simulink model "Experiment_AERO_pitch_channel_identification"  (Simulink 9.1)
settings: Solver=ode4  StartTime=0.0  StopTime=30  FixedStep=0.001  RelTol=1e-3  EnableMultiTasking=on
InitFcn:
  | Parameters_and_initial_conditions
values from neighbouring files (symbols this model uses):
  Dp = 0.0056    [Parameters_and_initial_conditions.m]    (also in quanser_aero_parameters.m = 0.0071116)
  Dy = 0.0220    (= 0.022)    [Parameters_and_initial_conditions.m]    (also in quanser_aero_parameters.m)
  Jp = J_body + 2*J_prop    (= 0.0218868648283)    [Parameters_and_initial_conditions.m]    (also in quanser_aero_parameters.m)
  Jy = J_body + 2*J_prop + J_yoke    (= 0.0219920648283)    [Parameters_and_initial_conditions.m]    (also in quanser_aero_parameters.m)
  Kpp = 10.9e-04    (= 0.00109)    [Parameters_and_initial_conditions.m]    (also in quanser_aero_parameters.m = 0.0011)
  Kpy = 0.0021    [Parameters_and_initial_conditions.m]    (also in quanser_aero_parameters.m)
  Ksp = 0.09    [Parameters_and_initial_conditions.m]    (also in quanser_aero_parameters.m = 0.037463)
  Kyp = -0.0027    [Parameters_and_initial_conditions.m]    (also in quanser_aero_parameters.m)
  Kyy = 0.0022    [Parameters_and_initial_conditions.m]    (also in quanser_aero_parameters.m)
  PitchAxisEnable = 1    [Parameters_and_initial_conditions.m]
  PitchMotorEnable = 1    [Parameters_and_initial_conditions.m]
  psi_dot_initial = 0.0    (= 0)    [Parameters_and_initial_conditions.m]
  psi_initial = 0.0    (= 0)    [Parameters_and_initial_conditions.m]
  theta_dot_initial = 0.0    (= 0)    [Parameters_and_initial_conditions.m]
  theta_initial = 0.0    (= 0)    [Parameters_and_initial_conditions.m]
  YawAxisEnable = 0    [Parameters_and_initial_conditions.m]
  YawMotorEnable = 0    [Parameters_and_initial_conditions.m]
libraries: quarc_library x7, simulink_extras x5, quanser_aero x1
settings Model: Creator=MLevis  LastModifiedBy=DELL  SimulationMode=external  ExtModeTrigDuration=5000
settings SolverCC: PositivePriorityOrder=on
settings DataIOCC: LimitDataPoints=on
settings DebuggingCC: UnderspecifiedInitializationDetection=Simplified  MergeDetectMultiDrivingBlocksExec=error  SolverPrmCheckMsg=warning
settings RTWCC: SystemTargetFile=quarc_win64.tlc  TemplateMakefile=quarc_default_tmf  Description=QUARC Win64 Target
settings STFCustomTargetCC: TargetPreCompLibLocation=C:\PROGRA~3\QUARC\lib\2018a\win64\release  ConcurrentExecutionCompliant=on  GeneratePreprocessorConditionals=Disable all  SystemTargetFile=quarc_win64.tlc
settings GRTTargetCC: TargetPreCompLibLocation=C:\PROGRA~3\QUARC\lib\2018a\win64\release  ParMdlRefBuildCompliant=off  CompOptLevelCompliant=off  GeneratePreprocessorConditionals=Disable all  MatFileLogging=off  CPPClassGenCompliant=off  UseToolchainInfoCompliant=off  ExtMode=on  ExtModeMexFile=quarc_comm
settings ConfigComp: CovSFcnEnable=off

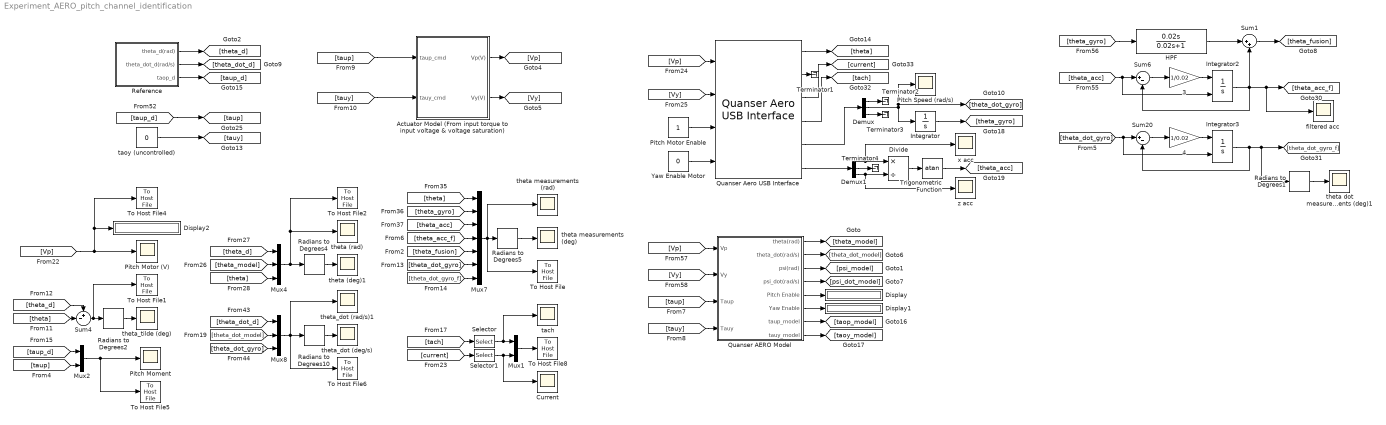
== system Experiment_AERO_pitch_channel_identification ==
  " 3" : Gain  Gain=1/0.02
  " 4" : Gain  Gain=1/0.02
  Actuator Model (From input torque to input voltage & voltage saturation) : Subsystem
  Current : Scope
  Demux : Demux  Outputs=3
  Demux1 : Demux  Outputs=3
  Display : Display
  Display1 : Display
  Display2 : Display
  Divide : Product  Inputs=*/
  HPF : TransferFcn  Numerator=[0.02 0]  Denominator=[0.02 1]
  Integrator : Integrator
  Integrator2 : Integrator  InitialConditionSource=external
  Integrator3 : Integrator  InitialConditionSource=external
  Mux1 : Mux  Inputs=2
  Mux2 : Mux  Inputs=2
  Mux4 : Mux  Inputs=3
  Mux7 : Mux  Inputs=7
  Mux8 : Mux  Inputs=3
  Pitch Moment : Scope
  Pitch Motor (V) : Scope
  Pitch Motor Enable : Constant
  Pitch Speed (rad/s) : Scope
  Quanser AERO Model : Subsystem
  Quanser Aero USB Interface : quanser_aero/Quanser Aero USB Interface
  Radians to Degrees{1..2,4..5,10} (5 alike) : simulink_extras/Transformations/Radians to Degrees
  Reference : Subsystem
  Selector : Selector  InputPortWidth=2  IndexOptions=Index vector (dialog)  Indices=[1]  OutputSizes=1
  Selector1 : Selector  InputPortWidth=2  IndexOptions=Index vector (dialog)  Indices=[1]  OutputSizes=1
  Sum1 : Sum  Inputs=|++
  Sum20 : Sum  Inputs=|+-
  Sum4 : Sum  Inputs=+-|
  Sum6 : Sum  Inputs=|+-
  Terminator{1..4} (4 alike) : Terminator
  To Host File : quarc_library/Sinks/To Host/To Host File  file_name=Log_Sensor_Measurements.mat  variable_name=Log_Sensor_Measurements  decimation=1  sample_time=-1  file_format=MAT-file v.5  options=No header or footer  append=off  final_file_name=Log_Sensor_Measurements.mat  bitrate=2000000
  To Host File1 : quarc_library/Sinks/To Host/To Host File  file_name=Log_Tracking_Err.mat  variable_name=Log_Tracking_Err  decimation=1  sample_time=-1  file_format=MAT-file v.5  options=No header or footer  append=off  final_file_name=Log_Tracking_Err.mat  bitrate=2000000
  To Host File2 : quarc_library/Sinks/To Host/To Host File  file_name=Log_Theta_Response.mat  variable_name=Log_Theta_Response  decimation=1  sample_time=-1  file_format=MAT-file v.5  options=No header or footer  append=off  final_file_name=Log_Theta_Response.mat  bitrate=2000000
  To Host File4 : quarc_library/Sinks/To Host/To Host File  file_name=Log_Input_Voltage.mat  variable_name=Log_Input_Voltage  decimation=1  sample_time=-1  file_format=MAT-file v.5  options=No header or footer  append=off  final_file_name=Log_Input_Voltage.mat  bitrate=2000000
  To Host File5 : quarc_library/Sinks/To Host/To Host File  file_name=Log_Input_Torque.mat  variable_name=Log_Input_Torque  decimation=1  sample_time=-1  file_format=MAT-file v.5  options=No header or footer  append=off  final_file_name=Log_Input_Torque.mat  bitrate=2000000
  To Host File6 : quarc_library/Sinks/To Host/To Host File  file_name=Log_Theta_dot_Response.mat  variable_name=Log_Theta_dot_Response  decimation=1  sample_time=-1  file_format=MAT-file v.5  options=No header or footer  append=off  final_file_name=Log_Theta_dot_Response.mat  bitrate=2000000
  To Host File8 : quarc_library/Sinks/To Host/To Host File  file_name=Log_Tach_Current.mat  variable_name=Log_Tach_Current  decimation=1  sample_time=-1  file_format=MAT-file v.5  options=No header or footer  append=off  final_file_name=Log_Tach_Current.mat  bitrate=2000000
  Trigonometric Function : Trigonometry  Operator=atan
  Yaw Enable Motor : Constant  Value=0
  filtered acc : Scope
  tach : Scope
  taoy (uncontrolled) : Constant  Value=0
  theta (deg)1 : Scope
  theta (rad) : Scope
  theta dot measurements (deg)1 : Scope
  theta measurements (deg) : Scope
  theta measurements (rad) : Scope
  theta_dot (deg/s) : Scope
  theta_dot (rad/s)1 : Scope
  theta_tilde (deg) : Scope
  x acc : Scope
  z acc : Scope
  wires:
  Quanser AERO Model/3(psi(rad)) -> [psi_model]
  Quanser AERO Model/1(theta(rad)) -> [theta_model]
  Reference/1(theta_d(rad)) -> [theta_d]
  Quanser AERO Model/2(theta_dot(rad/s)) -> [theta_dot_model]
  Quanser AERO Model/4(psi_dot(rad/s)) -> [psi_dot_model]
  Quanser AERO Model/5(Pitch Enable) -> Display/1
  Quanser AERO Model/6(Yaw Enable) -> Display1/1
  Actuator Model (From input torque to input voltage & voltage saturation)/1(Vp(V)) -> [Vp]
  Actuator Model (From input torque to input voltage & voltage saturation)/2(Vy(V)) -> [Vy]
  [tauy] -> Actuator Model (From input torque to input voltage & voltage saturation)/2(tauy_cmd)
  [taup] -> Actuator Model (From input torque to input voltage & voltage saturation)/1(taup_cmd)
  [theta_d] -> Sum4/1
  [theta] -> Sum4/2
  Sum4/1 -> To Host File1/1, Radians to Degrees2/1
  Radians to Degrees2/1 -> theta_tilde (deg)/1
  Reference/2(theta_dot_d(rad/s)) -> [theta_dot_d]
  Reference/3(taop_d) -> [taup_d]
  [taup] -> Mux2/2
  [taup_d] -> Mux2/1
  taoy (uncontrolled)/1 -> [tauy]
  [Vp] -> To Host File4/1, Display2/1, Pitch Motor (V)/1
  Quanser Aero USB Interface/5 -> Demux/1
  Yaw Enable Motor/1 -> Quanser Aero USB Interface/4
  Quanser Aero USB Interface/4 -> [tach]
  Quanser Aero USB Interface/1 -> [theta]
  Demux/3 -> Terminator3/1
  Pitch Motor Enable/1 -> Quanser Aero USB Interface/3
  Quanser Aero USB Interface/3 -> [current]
  [Vy] -> Quanser Aero USB Interface/2
  Demux/1 -> Terminator2/1
  Demux/2 -> Pitch Speed (rad/s)/1, [theta_dot_gyro], Integrator/1
  Quanser Aero USB Interface/2 -> Terminator1/1
  Quanser Aero USB Interface/6 -> Demux1/1
  [Vp] -> Quanser Aero USB Interface/1
  Radians to Degrees4/1 -> theta (deg)1/1
  [theta_model] -> Mux4/2
  [theta_d] -> Mux4/1
  [theta] -> Mux4/3
  Quanser AERO Model/7(taup_model) -> [taop_model]
  Mux2/1 -> To Host File5/1, Pitch Moment/1
  Quanser AERO Model/8(tauy_model) -> [taoy_model]
  Integrator/1 -> [theta_gyro]
  [theta] -> Mux7/1
  Demux1/1 -> Divide/1, x acc/1
  Demux1/2 -> Terminator4/1
  Demux1/3 -> Divide/2, z acc/1
  Divide/1 -> Trigonometric Function/1
  Trigonometric Function/1 -> [theta_acc]
  [theta_gyro] -> Mux7/2
  [theta_acc] -> Mux7/3
  Radians to Degrees5/1 -> theta measurements (deg)/1
  Radians to Degrees10/1 -> theta_dot (deg/s)/1
  [theta_dot_model] -> Mux8/2
  Mux8/1 -> theta_dot (rad/s)1/1, To Host File6/1, Radians to Degrees10/1
  [theta_dot_gyro] -> Mux8/3
  [theta_dot_d] -> Mux8/1
  [theta_gyro] -> HPF/1
  HPF/1 -> Sum1/1
  Sum1/1 -> [theta_fusion]
  [theta_acc_f] -> Mux7/4
  Mux7/1 -> theta measurements (rad)/1, To Host File/1, Radians to Degrees5/1
  [taup] -> Quanser AERO Model/3(Taup)
  [tauy] -> Quanser AERO Model/4(Tauy)
  [Vp] -> Quanser AERO Model/1(Vp)
  [Vy] -> Quanser AERO Model/2(Vy)
  [taup_d] -> [taup]
  Mux4/1 -> Radians to Degrees4/1, To Host File2/1, theta (rad)/1
  Integrator2/1 -> Sum1/2, Sum6/2, filtered acc/1, [theta_acc_f]
  " 3"/1 -> Integrator2/1
  Sum6/1 -> " 3"/1
  [theta_acc] -> Integrator2/2, Sum6/1
  [theta_fusion] -> Mux7/5
  [theta_dot_gyro] -> Integrator3/2, Sum20/1
  Sum20/1 -> " 4"/1
  " 4"/1 -> Integrator3/1
  Integrator3/1 -> Radians to Degrees1/1, [theta_dot_gyro_f], Sum20/2
  Radians to Degrees1/1 -> theta dot measurements (deg)1/1
  [theta_dot_gyro] -> Mux7/6
  [theta_dot_gyro_f] -> Mux7/7
  [tach] -> Selector/1
  Mux1/1 -> To Host File8/1
  [current] -> Selector1/1
  Selector/1 -> tach/1, Mux1/1
  Selector1/1 -> Current/1, Mux1/2

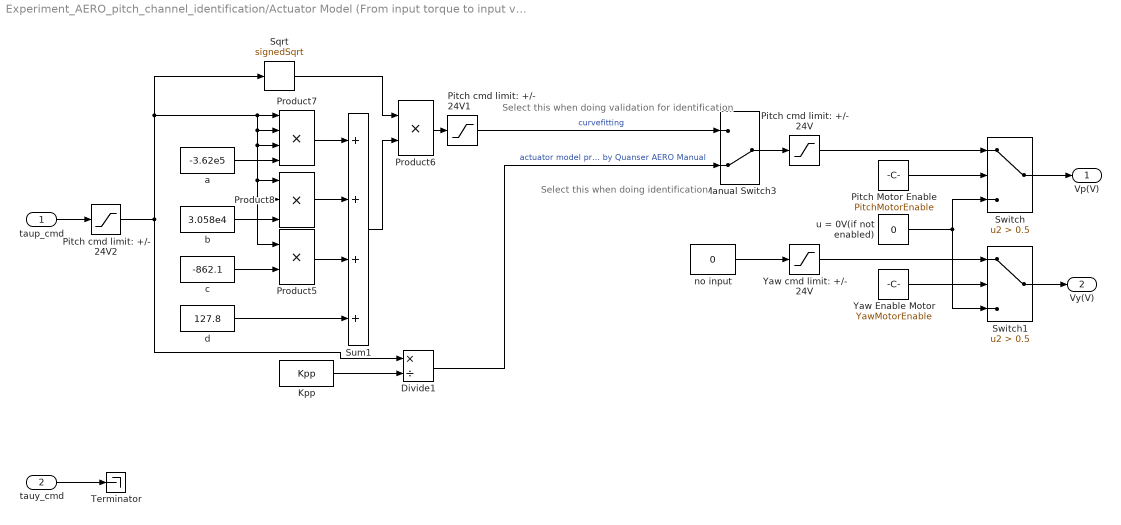
== system Experiment_AERO_pitch_channel_identification/Actuator Model (From input torque to input voltage & voltage saturation) ==
  note: Select this when doing identification
  note: Select this when doing validation for identification
  taup_cmd : Inport
  tauy_cmd : Inport  Port=2
  Divide1 : Product  Inputs=*/
  Kpp : Constant  Value=Kpp
  Manual Switch3 : ManualSwitch  CurrentSetting=0
  Pitch Motor Enable : Constant  Value=PitchMotorEnable
  Pitch cmd limit: +/- 24V : Saturate  UpperLimit=24  LowerLimit=-24
  Pitch cmd limit: +/- 24V1 : Saturate  UpperLimit=24  LowerLimit=0
  Pitch cmd limit: +/- 24V2 : Saturate  UpperLimit=0.05  LowerLimit=0
  Product5 : Product
  Product6 : Product
  Product7 : Product  Inputs=4
  Product8 : Product  Inputs=3
  Sqrt : Sqrt  Operator=signedSqrt  SaturateOnIntegerOverflow=on
  Sum1 : Sum  Inputs=++++
  Switch : Switch  Criteria=u2 > Threshold  Threshold=0.5
  Switch1 : Switch  Criteria=u2 > Threshold  Threshold=0.5
  Terminator : Terminator
  Yaw Enable Motor : Constant  Value=YawMotorEnable
  Yaw cmd limit: +/- 24V : Saturate  UpperLimit=24  LowerLimit=-24
  a : Constant  Value=-3.62e5
  b : Constant  Value=3.058e4
  c : Constant  Value=-862.1
  d : Constant  Value=127.8
  no input : Constant  Value=0
  u = 0V(if not enabled) : Constant  Value=0
  Vp(V) : Outport
  Vy(V) : Outport  Port=2
  wires:
  Pitch Motor Enable/1 -> Switch/2
  Yaw Enable Motor/1 -> Switch1/2
  Switch/1 -> Vp(V)/1
  Switch1/1 -> Vy(V)/1
  Yaw cmd limit: +/- 24V/1 -> Switch1/1
  Pitch cmd limit: +/- 24V/1 -> Switch/1
  u = 0V(if not enabled)/1 -> Switch1/3, Switch/3
  tauy_cmd/1 -> Terminator/1
  no input/1 -> Yaw cmd limit: +/- 24V/1
  Kpp/1 -> Divide1/2
  Manual Switch3/1 -> Pitch cmd limit: +/- 24V/1
  a/1 -> Product7/4
  b/1 -> Product8/3
  Sum1/1 -> Product6/2
  Sqrt/1 -> Product6/1
  Product6/1 -> Pitch cmd limit: +/- 24V1/1
  Divide1/1 -> Manual Switch3/2  "actuator model provided by Quanser AERO Manual"
  d/1 -> Sum1/4
  Product7/1 -> Sum1/1
  Product8/1 -> Sum1/2
  Product5/1 -> Sum1/3
  c/1 -> Product5/2
  taup_cmd/1 -> Pitch cmd limit: +/- 24V2/1
  Pitch cmd limit: +/- 24V1/1 -> Manual Switch3/1  "curvefitting"
  Pitch cmd limit: +/- 24V2/1 -> Sqrt/1, Product7/1, Product7/2, Product7/3, Product8/1, Product8/2, Product5/1, Divide1/1

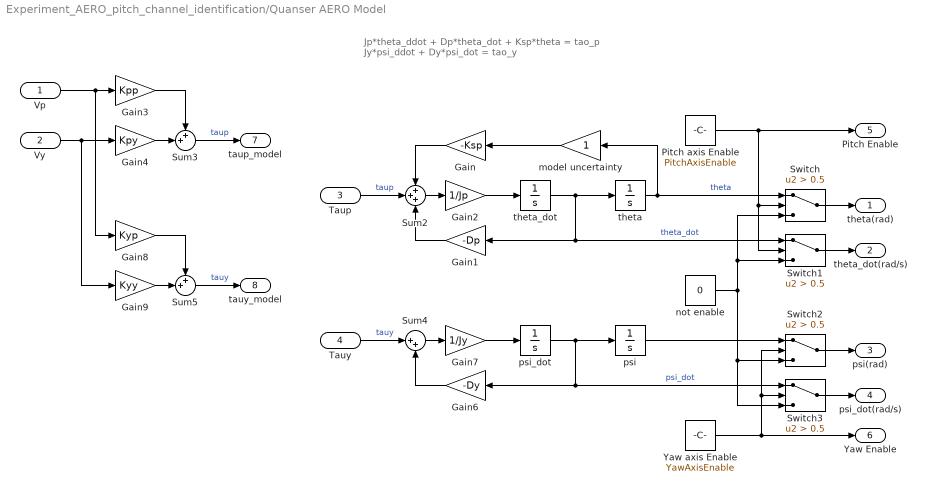
== system Experiment_AERO_pitch_channel_identification/Quanser AERO Model ==
  note: Jp*theta_ddot + Dp*theta_dot + Ksp*theta = tao_p
      | Jy*psi_ddot + Dy*psi_dot = tao_y
  Vp : Inport
  Vy : Inport  Port=2
  Taup : Inport  Port=3
  Tauy : Inport  Port=4
  Gain : Gain  Gain=-Ksp
  Gain1 : Gain  Gain=-Dp
  Gain2 : Gain  Gain=1/Jp
  Gain3 : Gain  Gain=Kpp
  Gain4 : Gain  Gain=Kpy
  Gain6 : Gain  Gain=-Dy
  Gain7 : Gain  Gain=1/Jy
  Gain8 : Gain  Gain=Kyp
  Gain9 : Gain  Gain=Kyy
  Pitch axis Enable : Constant  Value=PitchAxisEnable
  Sum2 : Sum  Inputs=+++
  Sum3 : Sum  Inputs=++|
  Sum4 : Sum  Inputs=|++
  Sum5 : Sum  Inputs=++|
  Switch{,1..3} (4 alike) : Switch  Criteria=u2 > Threshold  Threshold=0.5
  Yaw axis Enable : Constant  Value=YawAxisEnable
  model uncertainty : Gain
  not enable : Constant  Value=0
  psi : Integrator  InitialCondition=psi_initial
  psi_dot : Integrator  InitialCondition=psi_dot_initial
  theta : Integrator  InitialCondition=theta_initial
  theta_dot : Integrator  InitialCondition=theta_dot_initial
  theta(rad) : Outport
  theta_dot(rad/s) : Outport  Port=2
  psi(rad) : Outport  Port=3
  psi_dot(rad/s) : Outport  Port=4
  Pitch Enable : Outport  Port=5
  Yaw Enable : Outport  Port=6
  taup_model : Outport  Port=7
  tauy_model : Outport  Port=8
  wires:
  theta_dot/1 -> Gain1/1, Switch1/1, theta/1  "theta_dot"
  theta/1 -> Switch/1, model uncertainty/1  "theta"
  Taup/1 -> Sum2/2  "taup"
  Gain/1 -> Sum2/1
  Sum2/1 -> Gain2/1
  Gain2/1 -> theta_dot/1
  Gain3/1 -> Sum3/1
  Gain4/1 -> Sum3/2
  psi_dot/1 -> psi/1, Gain6/1, Switch3/1  "psi_dot"
  psi/1 -> Switch2/1
  Tauy/1 -> Sum4/1  "tauy"
  Sum4/1 -> Gain7/1
  Gain7/1 -> psi_dot/1
  Gain8/1 -> Sum5/1
  Gain9/1 -> Sum5/2
  Vp/1 -> Gain8/1, Gain3/1
  Vy/1 -> Gain9/1, Gain4/1
  Gain6/1 -> Sum4/2
  Pitch axis Enable/1 -> Pitch Enable/1, Switch1/2, Switch/2
  Switch/1 -> theta(rad)/1
  Switch1/1 -> theta_dot(rad/s)/1
  not enable/1 -> Switch1/3, Switch/3, Switch3/3, Switch2/3
  Switch2/1 -> psi(rad)/1
  Switch3/1 -> psi_dot(rad/s)/1
  Yaw axis Enable/1 -> Yaw Enable/1, Switch2/2, Switch3/2
  model uncertainty/1 -> Gain/1
  Gain1/1 -> Sum2/3
  Sum3/1 -> taup_model/1  "taup"
  Sum5/1 -> tauy_model/1  "tauy"

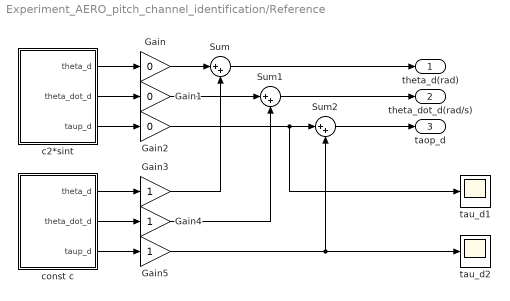
== system Experiment_AERO_pitch_channel_identification/Reference ==
  Gain : Gain  Gain=0
  Gain1 : Gain  Gain=0
  Gain2 : Gain  Gain=0
  Gain3 : Gain
  Gain4 : Gain
  Gain5 : Gain
  Sum : Sum  Inputs=|++
  Sum1 : Sum  Inputs=|++
  Sum2 : Sum  Inputs=|++
  c2*sint : Subsystem
  const c : Subsystem
  tau_d1 : Scope
  tau_d2 : Scope
  theta_d(rad) : Outport
  theta_dot_d(rad/s) : Outport  Port=2
  taop_d : Outport  Port=3
  wires:
  Sum1/1 -> theta_dot_d(rad/s)/1
  Sum2/1 -> taop_d/1
  Sum/1 -> theta_d(rad)/1
  c2*sint/1(theta_d) -> Gain/1
  const c/1(theta_d) -> Gain3/1
  c2*sint/2(theta_dot_d) -> Gain1/1
  const c/2(theta_dot_d) -> Gain4/1
  c2*sint/3(taup_d) -> Gain2/1
  const c/3(taup_d) -> Gain5/1
  Gain/1 -> Sum/1
  Gain1/1 -> Sum1/1
  Gain2/1 -> tau_d1/1, Sum2/1
  Gain4/1 -> Sum1/2
  Gain5/1 -> Sum2/2, tau_d2/1
  Gain3/1 -> Sum/2

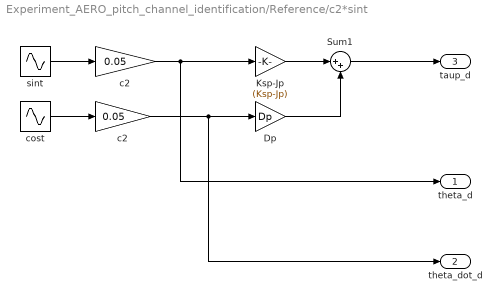
== system Experiment_AERO_pitch_channel_identification/Reference/c2*sint ==
  Dp : Gain  Gain=Dp
  Ksp-Jp : Gain  Gain=(Ksp-Jp)
  Sum1 : Sum  Inputs=|++
  c2 : Gain  Gain=0.05
  "c2 " : Gain  Gain=0.05
  cost : Sin  Phase=pi/2  SampleTime=0
  sint : Sin  SampleTime=0
  theta_d : Outport
  theta_dot_d : Outport  Port=2
  taup_d : Outport  Port=3
  wires:
  Dp/1 -> Sum1/2
  Ksp-Jp/1 -> Sum1/1
  sint/1 -> c2/1
  cost/1 -> "c2 "/1
  c2/1 -> theta_d/1, Ksp-Jp/1
  "c2 "/1 -> theta_dot_d/1, Dp/1
  Sum1/1 -> taup_d/1

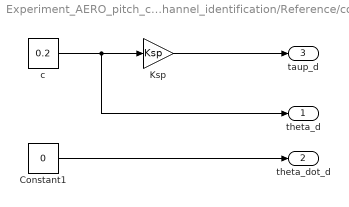
== system Experiment_AERO_pitch_channel_identification/Reference/const c ==
  Constant1 : Constant  Value=0
  Ksp : Gain  Gain=Ksp
  c : Constant  Value=0.2
  theta_d : Outport
  theta_dot_d : Outport  Port=2
  taup_d : Outport  Port=3
  wires:
  Ksp/1 -> taup_d/1
  c/1 -> theta_d/1, Ksp/1
  Constant1/1 -> theta_dot_d/1
